simulink model "DC_pos_AN"  (R2024a)
settings: Solver=ode5  StartTime=0.0  StopTime=60  FixedStep=0.01  RelTol=1e-3  EnableMultiTasking=on
undefined symbols (not defined in the file): sigbuilder_block
libraries: fuzblock x1
settings Model: Creator=DELL PC  LastModifiedBy=DELL PC
settings SolverCC: AlgebraicLoopSolver=TrustRegion  AutoInsertRateTranBlk=on
settings DataIOCC: ReturnWorkspaceOutputs=off
settings OptimizationCC: LifeSpan=inf
settings DebuggingCC: UnconnectedInputMsg=warning  UnconnectedOutputMsg=warning  UnconnectedLineMsg=warning  SFUnexpectedBacktrackingDiag=warning  SFNoUnconditionalDefaultTransitionDiag=warning  ArithmeticOperatorsInVariantConditions=warning
settings ModelReferenceCC: EnableRefExpFcnMdlSchedulingChecks=on
settings SFSimCC: SimUseLocalCustomCode=off  CustomCodeUndefinedFunction=UseInterfaceOnly
settings RTWCC: RTWUseLocalCustomCode=off  GPUComputeCapability=3.5
settings CodeAppCC: StateflowObjectComments=on
settings GRTTargetCC: TargetLangStandard=C89/C90 (ANSI)
settings ConfigComp: CovMetricSettings=dw  CovSaveCumulativeToWorkspaceVar=on  CovSaveSingleToWorkspaceVar=on  CovExternalEMLEnable=off

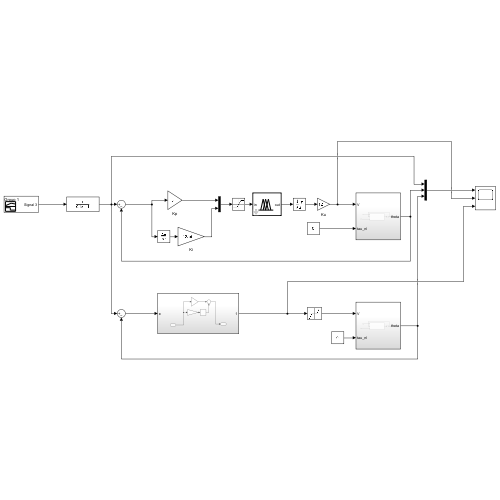
[thumbnail: Simulink's stored preview of the top-level diagram]
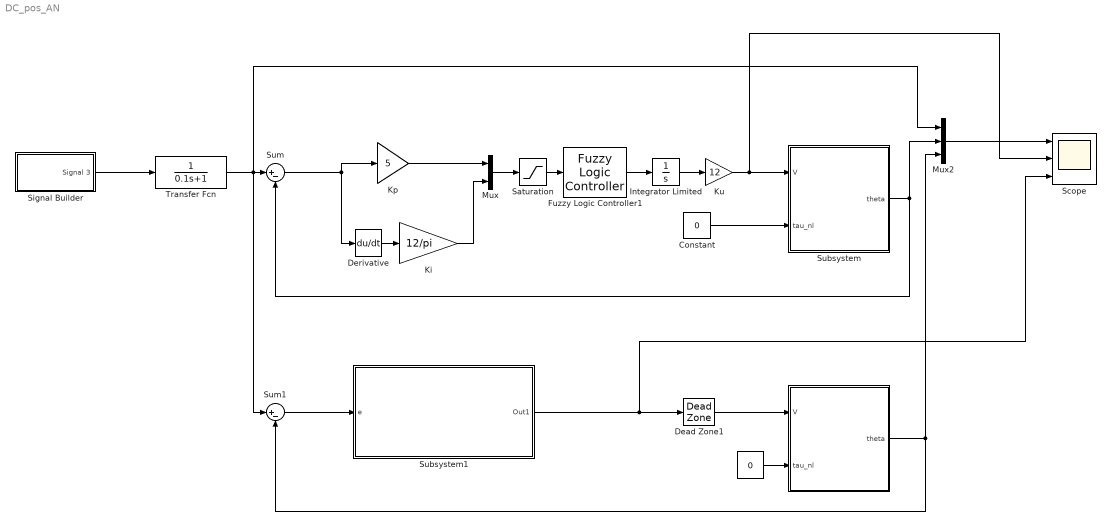
== system DC_pos_AN ==
  " " : Subsystem
  "  " : Constant  Value=0
  Constant : Constant  Value=0
  Dead Zone1 : DeadZone  LowerValue=-0.05  UpperValue=0.05
  Derivative : Derivative
  Fuzzy Logic Controller1 : fuzblock/Fuzzy Logic  Controller  FIS='DCVelMamdani3.fis'  OutputSampleNumber=101  DataType=double  FuzzifiedInputs=off  RuleFiringStrengths=off  RuleOutputs=off  AggregatedOutputs=off  SimulateUsing=Interpreted execution  OutOfRangeInputValueMessage=warning  NoRuleFiredMessage=warning  EmptyOutputFuzzySetMessage=warning
  Integrator Limited : Integrator  LimitOutput=on  UpperSaturationLimit=1  LowerSaturationLimit=-1
  Ki : Gain  Gain=12/pi
  "Kp " : Gain  Gain=5
  "Ku " : Gain  Gain=12
  Mux : Mux  Inputs=2
  Mux2 : Mux  Inputs=3
  Saturation : Saturate  UpperLimit=1  LowerLimit=-1
  Scope : Scope  NumInputPorts=3
  Signal Builder : Subsystem  Tag=STV Subsys  LoadFcn=sigbuilder_block('load');  StartFcn=sigbuilder_block('start');  StopFcn=sigbuilder_block('stop');  ClipboardFcn=sigbuilder_block('clipboard');  mask(Sigbuilder block){tuvar=[0:10]}
      mask help: Simulink:masks:SigbuilderBlock_MD
      mask init:
      | if ~strcmp(get_param(bdroot(gcbh),'SimulationStatus'),'stopped') tuvar = sigbuilder_block('maskInit'); end
      settings: CopyFcn=sigbuilder_block('copy');  DeleteFcn=sigbuilder_block('delete');  ModelCloseFcn=sigbuilder_block('modelClose');  PreSaveFcn=sigbuilder_block('preSave');  PauseFcn=sigbuilder_block('pause');  ContinueFcn=sigbuilder_block('continue');  NameChangeFcn=sigbuilder_block('namechange');  OpenFcn=sigbuilder_block('open',[5.5 5.5 949 474.5 ]);  CloseFcn=sigbuilder_block('close');
      mask Display: plot(0, 0, 100, 100,[2, 2, 32, 32, 2], [68, 8, 8, 68, 68],[32, 2], [38, 38], [32, 19, 2],[53, 60, 44], [32, 17, 17, 2],[16, 16, 31, 31]);txt = getActiveGroup(gcbh);text(2, 100, txt,'verticalAlignment', 'top');
  Subsystem : Subsystem
  Subsystem1 : Subsystem
  Sum : Sum  Inputs=|+-
  Sum1 : Sum  Inputs=|+-
  Transfer Fcn : TransferFcn  Denominator="[0.1  1 ]"
  wires:
  Sum/1 -> Derivative/1, "Kp "/1
  Integrator Limited/1 -> "Ku "/1
  Mux2/1 -> Scope/1
  "Kp "/1 -> Mux/1
  Derivative/1 -> Ki/1
  Constant/1 -> Subsystem/2(tau_nl)
  Fuzzy Logic Controller1/1 -> Integrator Limited/1
  Mux/1 -> Saturation/1
  Saturation/1 -> Fuzzy Logic Controller1/1
  Ki/1 -> Mux/2
  "Ku "/1 -> Scope/2, Subsystem/1(V)
  Subsystem/1(theta) -> Mux2/2, Sum/2
  Signal Builder/1(Signal 3) -> Transfer Fcn/1
  Transfer Fcn/1 -> Sum1/1, Mux2/1, Sum/1
  " "/1(theta) -> Sum1/2, Mux2/3
  Subsystem1/1(Out1) -> Scope/3, Dead Zone1/1
  Dead Zone1/1 -> " "/1(V)
  Sum1/1 -> Subsystem1/1(e)
  "  "/1 -> " "/2(tau_nl)

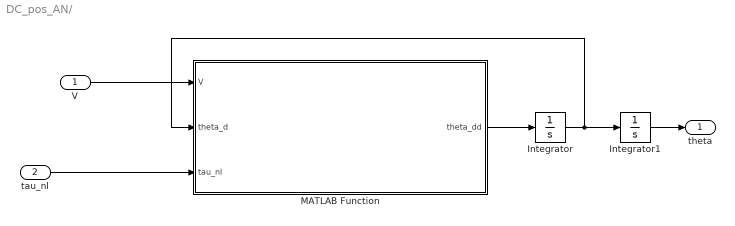
== system DC_pos_AN/  ==
  V : Inport
  tau_nl : Inport  Port=2
  Integrator : Integrator
  Integrator1 : Integrator
  MATLAB Function : MATLAB Function  TreatAsAtomicUnit=on
  theta : Outport
  wires:
  Integrator/1 -> Integrator1/1, MATLAB Function/2(theta_d)
  MATLAB Function/1(theta_dd) -> Integrator/1
  V/1 -> MATLAB Function/1(V)
  tau_nl/1 -> MATLAB Function/3(tau_nl)
  Integrator1/1 -> theta/1

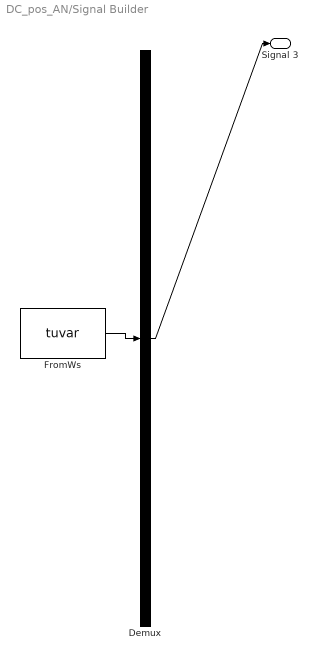
== system DC_pos_AN/Signal Builder ==
  Demux : Demux  Tag=STV Demux  Outputs=1
      settings: DisplayOption=none
  FromWs : FromWorkspace  Tag=STV FromWs  VariableName=tuvar
      SigBuilderData=|
      | common.afterFinalStr = 'Extrapolate'
      | common.sampleTime = 0
      | dataSet.timeRange = [0 60]
      | dataSet.name = 'Group 1'
      | sbobj.Groups.Name = 'Group 1'
      | sbobj.Groups.Signals.Name = 'Signal 3'
      | sbobj.Groups.Signals.XData = [0 10 10 20 20 30 30 40 40 50 50 60]
      | sbobj.Groups.Signals.YData = [1.57 1.57 0 0 -1.58 -1.58 0.78 0.78 0.02 0.02 3.14 3.14]
      | sbobj.Groups.TimeRange = [0 60]
  Signal 3 : Outport  Tag=STV Outport
  wires:
  FromWs/1 -> Demux/1
  Demux/1 -> Signal 3/1

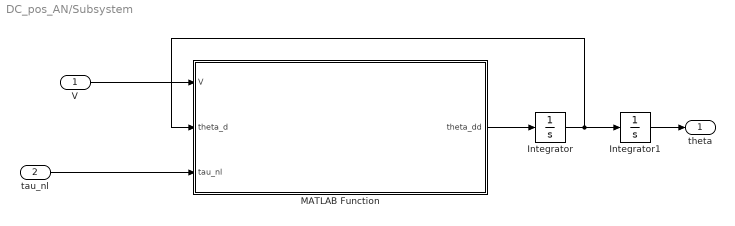
== system DC_pos_AN/Subsystem ==
  V : Inport
  tau_nl : Inport  Port=2
  Integrator : Integrator
  Integrator1 : Integrator
  MATLAB Function : MATLAB Function  TreatAsAtomicUnit=on
  theta : Outport
  wires:
  Integrator/1 -> Integrator1/1, MATLAB Function/2(theta_d)
  MATLAB Function/1(theta_dd) -> Integrator/1
  V/1 -> MATLAB Function/1(V)
  tau_nl/1 -> MATLAB Function/3(tau_nl)
  Integrator1/1 -> theta/1

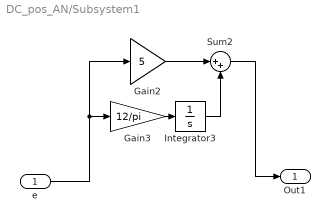
== system DC_pos_AN/Subsystem1 ==
  e : Inport
  Gain2 : Gain  Gain=5
  Gain3 : Gain  Gain=12/pi
  Integrator3 : Integrator
  Sum2 : Sum  Inputs=|++
  Out1 : Outport
  wires:
  e/1 -> Gain2/1, Gain3/1
  Gain3/1 -> Integrator3/1
  Integrator3/1 -> Sum2/2
  Gain2/1 -> Sum2/1
  Sum2/1 -> Out1/1

== matlab function DC_pos_AN/ /MATLAB Function ==
  data: V input; theta_d input; theta_dd output; tau_nl input
function theta_dd = motor_acceleration(V, theta_d, tau_nl)
    % Các thông số
    K = 0.2082   ;     % Hằng số mô-men (Nm/V)
    J = 0.001    ;   % Moment quán tính (kg.m^2)
    v = 0.0204  ;   % Hệ số ma sát nhớt (N.m.s)
    % Phương trình tính gia tốc góc
    theta_dd = (K*V - v*theta_d - tau_nl) / J;
end

== matlab function DC_pos_AN/Subsystem/MATLAB Function ==
  data: V input; theta_d input; theta_dd output; tau_nl input
function theta_dd = motor_acceleration(V, theta_d, tau_nl)
    % Các thông số
    K = 0.2082   ;     % Hằng số mô-men (Nm/V)
    J = 0.001 ;   % Moment quán tính (kg.m^2)
    v = 0.0204  ;   % Hệ số ma sát nhớt (N.m.s)
    % Phương trình tính gia tốc góc
    theta_dd = (K*V - v*theta_d - tau_nl) / J;
end
